simulink model "first_3phase_multilevel"  (R2015a)
settings: Solver=ode45  StartTime=0.02  StopTime=0.04  RelTol=1e-3
libraries: powerlib x95, powerlib_meascontrol x50, simulink x48, dspstat3 x2
(part 1 of 2)
settings Model: Creator=yahya  LastModifiedBy=Yahya

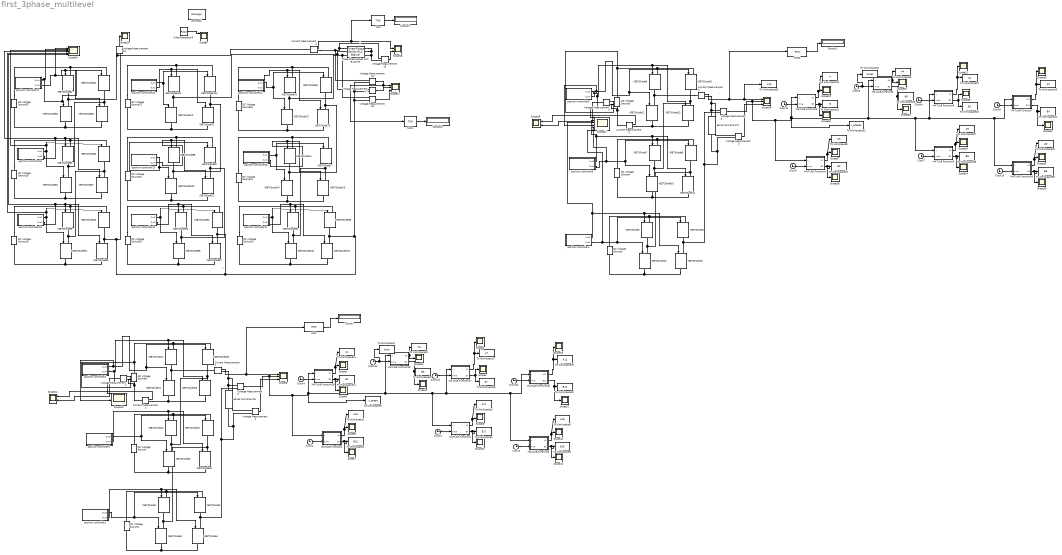
== system first_3phase_multilevel ==
  note: i
  note: n
  note: i
  note: i
  Clock{1..11,19..21} (14 alike) : Clock
  Current Measurement{1..5} (5 alike) : powerlib/Measurements/Current Measurement  PhasorSimulation=off  OutputType=Complex  PSBequivalent=0
  DC Voltage Source{1,3..5,7..8,18..26} (15 alike) : powerlib/Electrical Sources/DC Voltage Source  Amplitude=100  Measurements=None
  Display{,1..3} (4 alike) : Display
  IGBT/Diode{1..16,22..29,69..104} (60 alike) : powerlib/Power Electronics/IGBT//Diode  Ron=1e-3  Rs=1e5  Cs=inf  Measurements=off
  MATLAB Function1 : MATLAB Function  TreatAsAtomicUnit=on
  MATLAB Function10 : MATLAB Function  TreatAsAtomicUnit=on
  MATLAB Function16 : MATLAB Function  TreatAsAtomicUnit=on
  MATLAB Function17 : MATLAB Function  TreatAsAtomicUnit=on
  MATLAB Function18 : MATLAB Function  TreatAsAtomicUnit=on
  MATLAB Function19 : MATLAB Function  TreatAsAtomicUnit=on
  MATLAB Function2 : MATLAB Function  TreatAsAtomicUnit=on
  MATLAB Function3 : MATLAB Function  TreatAsAtomicUnit=on
  MATLAB Function4 : MATLAB Function  TreatAsAtomicUnit=on
  MATLAB Function5 : MATLAB Function  TreatAsAtomicUnit=on
  MATLAB Function6 : MATLAB Function  TreatAsAtomicUnit=on
  MATLAB Function7 : MATLAB Function  TreatAsAtomicUnit=on
  MATLAB Function8 : MATLAB Function  TreatAsAtomicUnit=on
  MATLAB Function9 : MATLAB Function  TreatAsAtomicUnit=on
  Pulse Generator3 : DiscretePulseGenerator  PulseType=Time based  Amplitude=0.8  Period=0.00001  PulseWidth=50
  RMS : dspstat3/RMS  run=off  reset_popup=None  InputProcessing=Columns as channels (frame based)  directionMode=Each column  dimension=1  treatSBRowAsCol=off
  RMS1 : dspstat3/RMS  run=off  reset_popup=None  InputProcessing=Columns as channels (frame based)  directionMode=Each column  dimension=1  treatSBRowAsCol=off
  Scope{1..4,6..8,10..12,15,19..26,29..35,37..39} (29 alike) : Scope
      Scope1 settings: TimeRange=0.2  YMin=190  YMax=400  SaveName=ScopeData6
      Scope10 settings: TimeRange=0.2  YMin=190  YMax=400  SaveName=ScopeData12
      Scope11 settings: TimeRange=0.2  YMin=190  YMax=400  SaveName=ScopeData14
      Scope12 settings: TimeRange=0.2  YMin=190  YMax=400  SaveName=ScopeData24
      Scope15 settings: TimeRange=0.2  YMin=190  YMax=400  SaveName=ScopeData27
      Scope19 settings: SaveName=ScopeData17
      Scope2 settings: TimeRange=0.2  YMin=190  YMax=400  SaveName=ScopeData7
      Scope20 settings: TimeRange=0.2  YMin=190  YMax=400  SaveName=ScopeData20
      Scope21 settings: TimeRange=0.2  YMin=190  YMax=400  SaveName=ScopeData21
      Scope22 settings: TimeRange=0.2  YMin=190  YMax=400  SaveName=ScopeData22
      Scope23 settings: TimeRange=0.2  YMin=190  YMax=400  SaveName=ScopeData23
      Scope24 settings: TimeRange=0.2  YMin=190  YMax=400  SaveName=ScopeData28
      Scope25 settings: TimeRange=0.2  YMin=190  YMax=400  SaveName=ScopeData29
      Scope26 settings: TimeRange=0.2  YMin=190  YMax=400  SaveName=ScopeData30
      Scope29 settings: TimeRange=0.2  YMin=190  YMax=400  SaveName=ScopeData33
      Scope3 settings: TimeRange=0.2  YMin=190  YMax=400  SaveName=ScopeData9
      Scope30 settings: TimeRange=0.2  YMin=190  YMax=400  SaveName=ScopeData34
      Scope31 settings: TimeRange=0.2  YMin=190  YMax=400  SaveName=ScopeData35
      Scope32 settings: TimeRange=0.2  YMin=190  YMax=400  SaveName=ScopeData36
      Scope33 settings: TimeRange=0.2  YMin=190  YMax=400  SaveName=ScopeData37
      Scope34 settings: TimeRange=0.2  YMin=190  YMax=400  SaveName=ScopeData38
      Scope35 settings: TimeRange=0.2  YMin=190  YMax=400  SaveName=ScopeData39
      Scope37 settings: TimeRange=0.2  YMin=190  YMax=400  SaveName=ScopeData41
      Scope38 settings: TimeRange=0.2  YMin=190  YMax=400  SaveName=ScopeData42
      Scope39 settings: TimeRange=0.2  YMin=190  YMax=400  SaveName=ScopeData43
      Scope4 settings: TimeRange=0.2  YMin=190  YMax=400  SaveName=ScopeData19
      Scope6 settings: TimeRange=0.2  YMin=190  YMax=400  SaveName=ScopeData10
      Scope7 settings: TimeRange=0.2  YMin=190  YMax=400  SaveName=ScopeData11
      Scope8 settings: TimeRange=0.2  YMin=190  YMax=400  SaveName=ScopeData13
  Scope13 : Scope  NumInputPorts=6
      settings: TimeRange=0.2  YMin=190~-5~-5~-5~-5~-5  YMax=400~5~5~5~5~5  SaveName=ScopeData25
  Scope14 : Scope  NumInputPorts=2
      settings: TimeRange=0.2  YMin=190~-5  YMax=400~5  SaveName=ScopeData26
  Scope16 : Scope  NumInputPorts=6
      settings: YMin=-5~-5~-5~-5~-5~-5  YMax=5~5~5~5~5~5  SaveName=ScopeData8
  Scope17 : Scope  NumInputPorts=3
      settings: TimeRange=0.02  YMin=-5~-5~-5  YMax=5~5~5  SaveName=ScopeData15
  Scope18 : Scope  NumInputPorts=2
      settings: TimeRange=1  YMin=-400~-400  YMax=400~400  SaveName=ScopeData16
  Scope27 : Scope  NumInputPorts=6
      settings: TimeRange=0.2  YMin=190~-5~-5~-5~-5~-5  YMax=400~5~5~5~5~5  SaveName=ScopeData31
  Scope28 : Scope  NumInputPorts=2
      settings: TimeRange=0.2  YMin=190~-5  YMax=400~5  SaveName=ScopeData32
  Scope36 : Scope  NumInputPorts=3
      settings: TimeRange=1  YMin=-400~-400~-5  YMax=400~400~5  SaveName=ScopeData40
  Scope5 : Scope  NumInputPorts=3
      settings: TimeRange=1  YMin=-400~-400~-5  YMax=400~400~5  SaveName=ScopeData3
  Scope9 : Scope  NumInputPorts=4
      settings: YMin=-5~-5~-5~-5  YMax=5~5~5~5  SaveName=ScopeData18
  Series RLC Branch1 : powerlib/Elements/Series RLC Branch  LConnTagsString=__new0  RConnTagsString=__new0  BranchType=R  Resistance=2000  Inductance=1e-5  SetiL0=off  InitialCurrent=0  Capacitance=1e-6  Setx0=off  InitialVoltage=0  Measurements=None
  Series RLC Branch5 : powerlib/Elements/Series RLC Branch  LConnTagsString=__new0  RConnTagsString=__new0  BranchType=R  Resistance=3000  Inductance=1e-5  SetiL0=off  InitialCurrent=0  Capacitance=1e-6  Setx0=off  InitialVoltage=0  Measurements=None
  THD : powerlib_meascontrol/Measurements/THD  Freq=50  Ts=0
  THD1 : powerlib_meascontrol/Measurements/THD  Freq=50  Ts=0
  Three-Phase Series RLC Branch3 : powerlib/Elements/Three-Phase Series RLC Branch  LConnTagsString=A|B|C  RConnTagsString=A|B|C  BranchType=RL  Resistance=1.405*2  Inductance=0.005839*2  Capacitance=1e-6  Measurements=Branch voltages
  To Workspace1 : ToWorkspace  VariableName=A13  SaveFormat=Timeseries  SampleTime=-1
  To Workspace10 : ToWorkspace  VariableName=A  SaveFormat=Timeseries  SampleTime=-1
  To Workspace11 : ToWorkspace  VariableName=A1  SaveFormat=Timeseries  SampleTime=-1
  To Workspace12 : ToWorkspace  VariableName=B  SaveFormat=Timeseries  SampleTime=-1
  To Workspace13 : ToWorkspace  VariableName=A2  SaveFormat=Timeseries  SampleTime=-1
  To Workspace14 : ToWorkspace  VariableName=B1  SaveFormat=Timeseries  SampleTime=-1
  To Workspace15 : ToWorkspace  VariableName=B2  SaveFormat=Timeseries  SampleTime=-1
  To Workspace16 : ToWorkspace  VariableName=A3  SaveFormat=Timeseries  SampleTime=-1
  To Workspace17 : ToWorkspace  VariableName=A7  SaveFormat=Timeseries  SampleTime=-1
  To Workspace18 : ToWorkspace  VariableName=B7  SaveFormat=Timeseries  SampleTime=-1
  To Workspace19 : ToWorkspace  VariableName=A11  SaveFormat=Timeseries  SampleTime=-1
  To Workspace2 : ToWorkspace  VariableName=B13  SaveFormat=Timeseries  SampleTime=-1
  To Workspace20 : ToWorkspace  VariableName=B11  SaveFormat=Timeseries  SampleTime=-1
  To Workspace21 : ToWorkspace  VariableName=A5  SaveFormat=Timeseries  SampleTime=-1
  To Workspace22 : ToWorkspace  VariableName=B5  SaveFormat=Timeseries  SampleTime=-1
  To Workspace23 : ToWorkspace  VariableName=B3  SaveFormat=Timeseries  SampleTime=-1
  To Workspace24 : ToWorkspace  VariableName=B4  SaveFormat=Timeseries  SampleTime=-1
  To Workspace25 : ToWorkspace  VariableName=A4  SaveFormat=Timeseries  SampleTime=-1
  To Workspace26 : ToWorkspace  VariableName=B6  SaveFormat=Timeseries  SampleTime=-1
  To Workspace27 : ToWorkspace  VariableName=A6  SaveFormat=Timeseries  SampleTime=-1
  To Workspace28 : ToWorkspace  VariableName=B8  SaveFormat=Timeseries  SampleTime=-1
  To Workspace29 : ToWorkspace  VariableName=A8  SaveFormat=Timeseries  SampleTime=-1
  To Workspace3 : ToWorkspace  VariableName=A17  SaveFormat=Timeseries  SampleTime=-1
  To Workspace30 : ToWorkspace  VariableName=B9  SaveFormat=Timeseries  SampleTime=-1
  To Workspace31 : ToWorkspace  VariableName=time1  SaveFormat=Timeseries  SampleTime=-1
  To Workspace32 : ToWorkspace  VariableName=v_phase1  SaveFormat=Timeseries  SampleTime=-1
  To Workspace33 : ToWorkspace  VariableName=A10  SaveFormat=Timeseries  SampleTime=-1
  To Workspace4 : ToWorkspace  VariableName=B17  SaveFormat=Timeseries  SampleTime=-1
  To Workspace5 : ToWorkspace  VariableName=A19  SaveFormat=Timeseries  SampleTime=-1
  To Workspace6 : ToWorkspace  VariableName=B19  SaveFormat=Timeseries  SampleTime=-1
  To Workspace7 : ToWorkspace  VariableName=time  SaveFormat=Timeseries  SampleTime=-1
  To Workspace8 : ToWorkspace  VariableName=v_phase  SaveFormat=Timeseries  SampleTime=-1
  To Workspace9 : ToWorkspace  VariableName=A9  SaveFormat=Timeseries  SampleTime=-1
  Voltage Measurement{1..6,15..19} (11 alike) : powerlib/Measurements/Voltage Measurement  PhasorSimulation=off  OutputType=Complex  PSBequivalent=0
  position controller1 : Subsystem
  position controller17 : Subsystem
  position controller18 : Subsystem
  position controller19 : Subsystem
  position controller2 : Subsystem
  position controller20 : Subsystem
  position controller21 : Subsystem
  position controller22 : Subsystem
  position controller23 : Subsystem
  position controller24 : Subsystem
  position controller25 : Subsystem
  position controller3 : Subsystem
  position controller4 : Subsystem
  position controller5 : Subsystem
  position controller6 : Subsystem
  powergui : powerlib/powergui  Priority=1  SimulationMode=Continuous  SolverType=Tustin/Backward Euler (TBE)  SampleTime=50e-6  frequency=60  SPID=off  DisableSnubberDevices=off  DisableRonSwitches=off  DisableVfSwitches=off  SwTol=0  DisplayEquations=off  Interpol=off  methode=off  Ts=100  FunctionMessages=off  echomessages=off  HookPort=off  EnableUseOfTLC=off  x0status=blocks  frequencyindice=0  Pbase=100e6  ErrMax=1e-4  Iterations=50  UnitsV=kV  UnitsW=MW  buscounter=0  RestoreLinks=warning  ResistiveCurrentMeasurement=off  Frange=[0:2:500]  Ylog=off  Xlog=on  ShowGrid=off  save=off  variable=ZData  structure=0  ZoomFFT=off  StartTime=0.0  cycles=1  DisplayStyle=1  fundamental=60  FreqAxis=off  MaxFrequency=1000  frequencyindicesteady=1  RmsSteady=1  display=off
  wires:
  position controller2/2(Out4) -> Scope13/1, IGBT/Diode28/1, IGBT/Diode24/1
  position controller2/1(Out3) -> Scope13/4, IGBT/Diode26/1, IGBT/Diode27/1
  position controller3/2(Out4) -> IGBT/Diode29/1, IGBT/Diode22/1
  position controller3/1(Out3) -> IGBT/Diode23/1, IGBT/Diode25/1
  Current Measurement1/1 -> RMS/1, Scope5/1
  Voltage Measurement4/1 -> Scope5/3
  position controller17/2(Out2) -> Scope16/1, IGBT/Diode86/1, IGBT/Diode82/1
  Pulse Generator3/1 -> Scope9/1
  Current Measurement4/1 -> THD/1, Scope18/1
  position controller17/1(Out1) -> Scope16/2, IGBT/Diode85/1, IGBT/Diode84/1
  position controller18/2(Out2) -> Scope16/4, IGBT/Diode87/1, IGBT/Diode69/1
  position controller18/1(Out1) -> IGBT/Diode83/1, Scope16/3, IGBT/Diode80/1
  position controller22/2(Out2) -> IGBT/Diode71/1, IGBT/Diode102/1
  position controller22/1(Out1) -> IGBT/Diode70/1, IGBT/Diode104/1
  position controller23/2(Out2) -> IGBT/Diode72/1, IGBT/Diode88/1
  position controller23/1(Out1) -> IGBT/Diode103/1, IGBT/Diode92/1
  position controller24/2(Out2) -> IGBT/Diode74/1, IGBT/Diode78/1
  position controller24/1(Out1) -> IGBT/Diode81/1, IGBT/Diode73/1
  position controller25/2(Out2) -> IGBT/Diode75/1, IGBT/Diode76/1
  position controller25/1(Out1) -> IGBT/Diode79/1, IGBT/Diode77/1
  Voltage Measurement19/1 -> Scope19/1
  Voltage Measurement15/1 -> Scope18/2
  Voltage Measurement16/1 -> Scope17/1, THD1/1
  Voltage Measurement17/1 -> Scope17/2
  Voltage Measurement18/1 -> Scope17/3
  position controller19/2(Out2) -> Scope16/6, IGBT/Diode93/1, IGBT/Diode89/1
  position controller19/1(Out1) -> IGBT/Diode91/1, Scope16/5, IGBT/Diode90/1
  position controller20/2(Out2) -> IGBT/Diode97/1, IGBT/Diode94/1
  position controller20/1(Out1) -> IGBT/Diode96/1, IGBT/Diode95/1
  position controller21/2(Out2) -> IGBT/Diode101/1, IGBT/Diode98/1
  position controller21/1(Out1) -> IGBT/Diode100/1, IGBT/Diode99/1
  position controller1/2(Out4) -> IGBT/Diode4/1, IGBT/Diode1/1
  position controller1/1(Out3) -> IGBT/Diode3/1, IGBT/Diode2/1
  Clock4/1 -> MATLAB Function16/2(time)
  MATLAB Function16/1(A1) -> To Workspace11/1, Scope2/1
  MATLAB Function16/2(B1) -> Scope3/1, To Workspace14/1
  Clock19/1 -> MATLAB Function17/2(time)
  MATLAB Function17/1(A7) -> Scope1/1, To Workspace17/1
  MATLAB Function17/2(B7) -> To Workspace18/1, Scope4/1
  Clock20/1 -> MATLAB Function18/2(time)
  MATLAB Function18/1(A11) -> Scope20/1, To Workspace19/1
  MATLAB Function18/2(B11) -> Scope21/1, To Workspace20/1
  MATLAB Function19/1(A5) -> Scope22/1, To Workspace21/1
  MATLAB Function19/2(B5) -> Scope23/1, To Workspace22/1
  Clock1/1 -> MATLAB Function1/2(time)
  MATLAB Function1/1(A1) -> To Workspace1/1, Scope6/1
  MATLAB Function1/2(B1) -> Scope7/1, To Workspace2/1
  Clock2/1 -> MATLAB Function2/2(time)
  MATLAB Function2/1(A1) -> To Workspace3/1, Scope8/1
  MATLAB Function2/2(B1) -> Scope10/1, To Workspace4/1
  Clock3/1 -> MATLAB Function3/2(time)
  MATLAB Function3/1(A1) -> To Workspace5/1, Scope12/1
  MATLAB Function3/2(B1) -> Scope11/1, To Workspace6/1
  Voltage Measurement5/1 -> MATLAB Function1/1(u), MATLAB Function2/1(u), MATLAB Function3/1(u), MATLAB Function18/1(u), MATLAB Function17/1(u), MATLAB Function19/1(u), To Workspace8/1, MATLAB Function16/1(u), Scope5/2
  Clock21/1 -> To Workspace7/1, MATLAB Function19/2(time)
  Current Measurement2/1 -> Scope14/1
  Voltage Measurement1/1 -> Scope14/2
  RMS/1 -> Display/1
  position controller5/1(Out3) -> Scope27/1, IGBT/Diode13/1, IGBT/Diode9/1
  position controller5/2(Out4) -> Scope27/4, IGBT/Diode11/1, IGBT/Diode12/1
  position controller6/1(Out3) -> Scope27/2, IGBT/Diode14/1, IGBT/Diode7/1
  position controller6/2(Out4) -> Scope27/5, IGBT/Diode8/1, IGBT/Diode10/1
  Current Measurement3/1 -> RMS1/1, To Workspace33/1, Scope36/1
  Voltage Measurement3/1 -> Scope36/3
  position controller4/1(Out3) -> Scope27/3, IGBT/Diode16/1, IGBT/Diode5/1
  position controller4/2(Out4) -> Scope27/6, IGBT/Diode15/1, IGBT/Diode6/1
  Clock11/1 -> MATLAB Function5/2(time)
  MATLAB Function5/1(A1) -> To Workspace10/1, Scope29/1
  MATLAB Function5/2(B1) -> Scope34/1, To Workspace12/1
  Clock6/1 -> MATLAB Function6/2(time)
  MATLAB Function6/1(A7) -> Scope15/1, To Workspace13/1
  MATLAB Function6/2(B7) -> To Workspace15/1, Scope35/1
  Clock8/1 -> MATLAB Function7/2(time)
  MATLAB Function7/1(A11) -> Scope30/1, To Workspace16/1
  MATLAB Function7/2(B11) -> Scope31/1, To Workspace24/1
  MATLAB Function8/1(A5) -> Scope32/1, To Workspace25/1
  MATLAB Function8/2(B5) -> Scope33/1, To Workspace26/1
  Clock5/1 -> MATLAB Function4/2(time)
  MATLAB Function4/1(A1) -> To Workspace9/1, Scope37/1
  MATLAB Function4/2(B1) -> Scope38/1, To Workspace23/1
  Clock7/1 -> MATLAB Function9/2(time)
  MATLAB Function9/1(A1) -> To Workspace27/1, Scope39/1
  MATLAB Function9/2(B1) -> Scope24/1, To Workspace28/1
  Clock10/1 -> MATLAB Function10/2(time)
  MATLAB Function10/1(A1) -> To Workspace29/1, Scope26/1
  MATLAB Function10/2(B1) -> Scope25/1, To Workspace30/1
  Voltage Measurement6/1 -> MATLAB Function4/1(u), MATLAB Function9/1(u), MATLAB Function10/1(u), MATLAB Function7/1(u), MATLAB Function6/1(u), MATLAB Function8/1(u), To Workspace32/1, MATLAB Function5/1(u), Scope36/2
  Clock9/1 -> To Workspace31/1, MATLAB Function8/2(time)
  Current Measurement5/1 -> Scope28/1
  Voltage Measurement2/1 -> Scope28/2
  RMS1/1 -> Display1/1
  THD/1 -> Display2/1
  THD1/1 -> Display3/1
  connections:
  IGBT/Diode26/LConn1 -- IGBT/Diode24/LConn1 -- DC Voltage Source8/RConn1 -- Voltage Measurement1/LConn2
  IGBT/Diode28/RConn1 -- Current Measurement2/RConn1 -- IGBT/Diode27/RConn1
  IGBT/Diode24/RConn1 -- IGBT/Diode27/LConn1 -- Current Measurement1/LConn1
  DC Voltage Source7/RConn1 -- IGBT/Diode23/LConn1 -- IGBT/Diode22/LConn1
  DC Voltage Source7/LConn1 -- IGBT/Diode29/RConn1 -- IGBT/Diode25/RConn1
  IGBT/Diode22/RConn1 -- IGBT/Diode25/LConn1 -- IGBT/Diode28/LConn1 -- IGBT/Diode26/RConn1
  IGBT/Diode3/LConn1 -- IGBT/Diode29/LConn1 -- IGBT/Diode23/RConn1 -- IGBT/Diode1/RConn1
  Voltage Measurement5/LConn1 -- Series RLC Branch5/LConn1 -- Voltage Measurement4/LConn1 -- Current Measurement1/RConn1
  DC Voltage Source25/RConn1 -- IGBT/Diode84/LConn1 -- IGBT/Diode82/LConn1
  DC Voltage Source25/LConn1 -- IGBT/Diode85/RConn1 -- IGBT/Diode86/RConn1
  IGBT/Diode84/RConn1 -- IGBT/Diode86/LConn1 -- IGBT/Diode69/RConn1 -- IGBT/Diode83/LConn1
  DC Voltage Source18/RConn1 -- IGBT/Diode80/LConn1 -- IGBT/Diode69/LConn1
  DC Voltage Source18/LConn1 -- IGBT/Diode87/RConn1 -- IGBT/Diode83/RConn1
  DC Voltage Source23/RConn1 -- IGBT/Diode104/LConn1 -- IGBT/Diode102/LConn1
  DC Voltage Source23/LConn1 -- IGBT/Diode71/RConn1 -- IGBT/Diode70/RConn1
  Voltage Measurement17/LConn1 -- Three-Phase Series RLC Branch3/LConn2 -- IGBT/Diode102/RConn1 -- IGBT/Diode70/LConn1
  IGBT/Diode92/LConn1 -- DC Voltage Source22/RConn1 -- IGBT/Diode88/LConn1
  DC Voltage Source22/LConn1 -- IGBT/Diode72/RConn1 -- IGBT/Diode103/RConn1
  IGBT/Diode88/RConn1 -- IGBT/Diode103/LConn1 -- IGBT/Diode71/LConn1 -- IGBT/Diode104/RConn1
  DC Voltage Source26/RConn1 -- IGBT/Diode81/LConn1 -- IGBT/Diode78/LConn1
  DC Voltage Source26/LConn1 -- IGBT/Diode74/RConn1 -- IGBT/Diode73/RConn1
  DC Voltage Source24/RConn1 -- IGBT/Diode77/LConn1 -- IGBT/Diode76/LConn1
  DC Voltage Source24/LConn1 -- IGBT/Diode75/RConn1 -- IGBT/Diode79/RConn1
  IGBT/Diode74/LConn1 -- IGBT/Diode81/RConn1 -- IGBT/Diode76/RConn1 -- IGBT/Diode79/LConn1
  IGBT/Diode73/LConn1 -- IGBT/Diode78/RConn1 -- Three-Phase Series RLC Branch3/LConn3 -- Voltage Measurement18/LConn1
  IGBT/Diode82/RConn1 -- IGBT/Diode85/LConn1 -- Current Measurement4/LConn1 -- Voltage Measurement19/LConn1
  Three-Phase Series RLC Branch3/LConn1 -- Voltage Measurement15/LConn1 -- Voltage Measurement16/LConn1 -- Current Measurement4/RConn1
  Three-Phase Series RLC Branch3/RConn1 -- Three-Phase Series RLC Branch3/RConn2 -- Three-Phase Series RLC Branch3/RConn3 -- Voltage Measurement15/LConn2
  IGBT/Diode89/RConn1 -- IGBT/Diode91/LConn1 -- IGBT/Diode80/RConn1 -- IGBT/Diode87/LConn1
  IGBT/Diode94/RConn1 -- IGBT/Diode96/LConn1 -- IGBT/Diode92/RConn1 -- IGBT/Diode72/LConn1
  IGBT/Diode98/RConn1 -- IGBT/Diode100/LConn1 -- IGBT/Diode77/RConn1 -- IGBT/Diode75/LConn1
  DC Voltage Source19/RConn1 -- IGBT/Diode90/LConn1 -- IGBT/Diode89/LConn1
  DC Voltage Source19/LConn1 -- IGBT/Diode93/RConn1 -- IGBT/Diode91/RConn1
  DC Voltage Source20/RConn1 -- IGBT/Diode95/LConn1 -- IGBT/Diode94/LConn1
  DC Voltage Source20/LConn1 -- IGBT/Diode97/RConn1 -- IGBT/Diode96/RConn1
  DC Voltage Source21/RConn1 -- IGBT/Diode99/LConn1 -- IGBT/Diode98/LConn1
  DC Voltage Source21/LConn1 -- IGBT/Diode101/RConn1 -- IGBT/Diode100/RConn1
  IGBT/Diode93/LConn1 -- IGBT/Diode90/RConn1 -- Voltage Measurement19/LConn2 -- Voltage Measurement16/LConn2 -- Voltage Measurement17/LConn2 -- Voltage Measurement18/LConn2 -- IGBT/Diode99/RConn1 -- IGBT/Diode101/LConn1 -- IGBT/Diode95/RConn1 -- IGBT/Diode97/LConn1
  IGBT/Diode1/LConn1 -- DC Voltage Source1/RConn1 -- IGBT/Diode2/LConn1
  IGBT/Diode3/RConn1 -- DC Voltage Source1/LConn1 -- IGBT/Diode4/RConn1
  Voltage Measurement4/LConn2 -- IGBT/Diode4/LConn1 -- IGBT/Diode2/RConn1 -- Voltage Measurement5/LConn2 -- Series RLC Branch5/RConn1
  DC Voltage Source8/LConn1 -- Current Measurement2/LConn1 -- Voltage Measurement1/LConn1
  IGBT/Diode9/LConn1 -- DC Voltage Source5/RConn1 -- Voltage Measurement2/LConn2 -- IGBT/Diode11/LConn1
  IGBT/Diode12/RConn1 -- IGBT/Diode13/RConn1 -- Current Measurement5/RConn1
  Current Measurement3/LConn1 -- IGBT/Diode9/RConn1 -- IGBT/Diode12/LConn1
  IGBT/Diode7/LConn1 -- DC Voltage Source4/RConn1 -- IGBT/Diode8/LConn1
  IGBT/Diode10/RConn1 -- DC Voltage Source4/LConn1 -- IGBT/Diode14/RConn1
  IGBT/Diode11/RConn1 -- IGBT/Diode13/LConn1 -- IGBT/Diode7/RConn1 -- IGBT/Diode10/LConn1
  IGBT/Diode5/RConn1 -- IGBT/Diode15/LConn1 -- IGBT/Diode14/LConn1 -- IGBT/Diode8/RConn1
  Current Measurement3/RConn1 -- Voltage Measurement3/LConn1 -- Voltage Measurement6/LConn1 -- Series RLC Branch1/LConn1
  IGBT/Diode6/LConn1 -- IGBT/Diode5/LConn1 -- DC Voltage Source3/RConn1
  IGBT/Diode16/RConn1 -- IGBT/Diode15/RConn1 -- DC Voltage Source3/LConn1
  Series RLC Branch1/RConn1 -- Voltage Measurement3/LConn2 -- IGBT/Diode16/LConn1 -- IGBT/Diode6/RConn1 -- Voltage Measurement6/LConn2
  Voltage Measurement2/LConn1 -- DC Voltage Source5/LConn1 -- Current Measurement5/LConn1

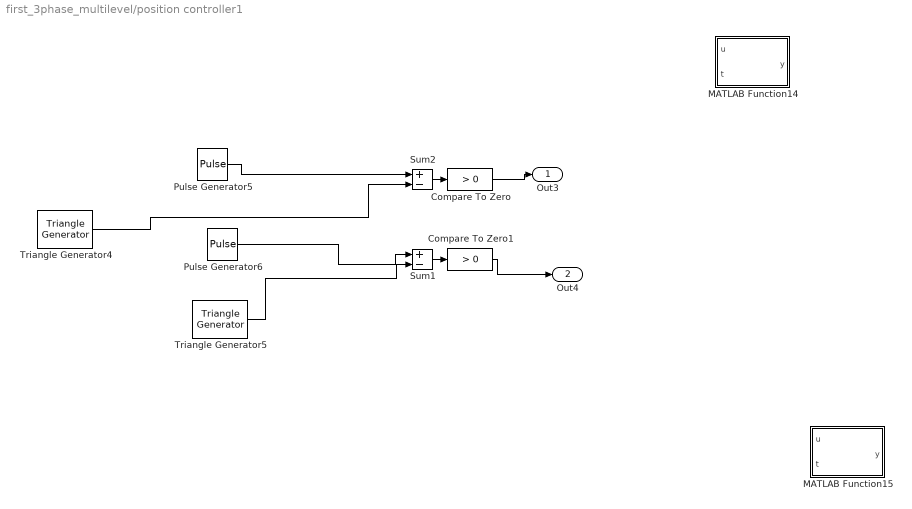
== system first_3phase_multilevel/position controller1 ==
  Compare To Zero : simulink/Logic and Bit Operations/Compare To Zero  relop=>  OutDataTypeStr=boolean  ZeroCross=off
  Compare To Zero1 : simulink/Logic and Bit Operations/Compare To Zero  relop=>  OutDataTypeStr=boolean  ZeroCross=off
  MATLAB Function14 : MATLAB Function  TreatAsAtomicUnit=on
  MATLAB Function15 : MATLAB Function  TreatAsAtomicUnit=on
  Pulse Generator5 : DiscretePulseGenerator  PulseType=Time based  Amplitude=0.138082553598467  Period=0.02  PulseWidth=50.001
  Pulse Generator6 : DiscretePulseGenerator  PulseType=Time based  Amplitude=0.138082553598467  Period=0.02  PulseWidth=50.001  PhaseDelay=0.01
  Sum1 : Sum  Inputs=+-  OutDataTypeStr=double
  Sum2 : Sum  Inputs=+-  OutDataTypeStr=double
  Triangle Generator4 : powerlib_meascontrol/Pulse & Signal Generators/Triangle Generator  Freq=50  Phase=90  Ts=0
  Triangle Generator5 : powerlib_meascontrol/Pulse & Signal Generators/Triangle Generator  Freq=50  Phase=90+180  Ts=0
  Out3 : Outport
  Out4 : Outport  Port=2
  wires:
  Compare To Zero/1 -> Out3/1
  Compare To Zero1/1 -> Out4/1
  Triangle Generator4/1 -> Sum2/2
  Sum2/1 -> Compare To Zero/1
  Sum1/1 -> Compare To Zero1/1
  Pulse Generator5/1 -> Sum2/1
  Pulse Generator6/1 -> Sum1/1
  Triangle Generator5/1 -> Sum1/2

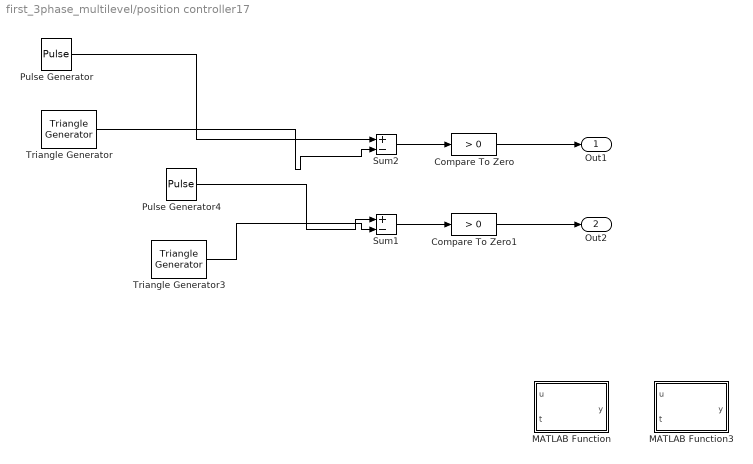
== system first_3phase_multilevel/position controller17 ==
  Compare To Zero : simulink/Logic and Bit Operations/Compare To Zero  relop=>  OutDataTypeStr=boolean  ZeroCross=off
  Compare To Zero1 : simulink/Logic and Bit Operations/Compare To Zero  relop=>  OutDataTypeStr=boolean  ZeroCross=off
  MATLAB Function : MATLAB Function  TreatAsAtomicUnit=on
  MATLAB Function3 : MATLAB Function  TreatAsAtomicUnit=on
  Pulse Generator : DiscretePulseGenerator  PulseType=Time based  Amplitude=0.9774  Period=0.02  PulseWidth=50
  Pulse Generator4 : DiscretePulseGenerator  PulseType=Time based  Amplitude=0.9774  Period=0.02  PulseWidth=50  PhaseDelay=0.01
  Sum1 : Sum  Inputs=+-  OutDataTypeStr=double
  Sum2 : Sum  Inputs=+-  OutDataTypeStr=double
  Triangle Generator : powerlib_meascontrol/Pulse & Signal Generators/Triangle Generator  Freq=50  Phase=90  Ts=0
  Triangle Generator3 : powerlib_meascontrol/Pulse & Signal Generators/Triangle Generator  Freq=50  Phase=90+180  Ts=0
  Out1 : Outport
  Out2 : Outport  Port=2
  wires:
  Compare To Zero/1 -> Out1/1
  Pulse Generator/1 -> Sum2/1
  Triangle Generator/1 -> Sum2/2
  Pulse Generator4/1 -> Sum1/1
  Triangle Generator3/1 -> Sum1/2
  Compare To Zero1/1 -> Out2/1
  Sum2/1 -> Compare To Zero/1
  Sum1/1 -> Compare To Zero1/1

== system first_3phase_multilevel/position controller18 ==
  Compare To Zero : simulink/Logic and Bit Operations/Compare To Zero  relop=>  OutDataTypeStr=boolean  ZeroCross=off
  Compare To Zero1 : simulink/Logic and Bit Operations/Compare To Zero  relop=>  OutDataTypeStr=boolean  ZeroCross=off
  Pulse Generator5 : DiscretePulseGenerator  PulseType=Time based  Amplitude=0.9502  Period=0.02  PulseWidth=50
  Pulse Generator6 : DiscretePulseGenerator  PulseType=Time based  Amplitude=0.9502  Period=0.02  PulseWidth=50  PhaseDelay=0.01
  Sum1 : Sum  Inputs=+-  OutDataTypeStr=double
  Sum2 : Sum  Inputs=+-  OutDataTypeStr=double
  Triangle Generator4 : powerlib_meascontrol/Pulse & Signal Generators/Triangle Generator  Freq=50  Phase=90  Ts=0
  Triangle Generator5 : powerlib_meascontrol/Pulse & Signal Generators/Triangle Generator  Freq=50  Phase=90+180  Ts=0
  Out1 : Outport
  Out2 : Outport  Port=2
  wires:
  Compare To Zero/1 -> Out1/1
  Compare To Zero1/1 -> Out2/1
  Pulse Generator5/1 -> Sum2/1
  Triangle Generator4/1 -> Sum2/2
  Pulse Generator6/1 -> Sum1/1
  Triangle Generator5/1 -> Sum1/2
  Sum2/1 -> Compare To Zero/1
  Sum1/1 -> Compare To Zero1/1

== system first_3phase_multilevel/position controller19 ==
  Compare To Zero : simulink/Logic and Bit Operations/Compare To Zero  relop=>  OutDataTypeStr=boolean  ZeroCross=off
  Compare To Zero1 : simulink/Logic and Bit Operations/Compare To Zero  relop=>  OutDataTypeStr=boolean  ZeroCross=off
  Pulse Generator5 : DiscretePulseGenerator  PulseType=Time based  Amplitude=0.5294  Period=0.02  PulseWidth=50
  Pulse Generator6 : DiscretePulseGenerator  PulseType=Time based  Amplitude=0.5294  Period=0.02  PulseWidth=50  PhaseDelay=0.01
  Sum1 : Sum  Inputs=+-  OutDataTypeStr=double
  Sum2 : Sum  Inputs=+-  OutDataTypeStr=double
  Triangle Generator4 : powerlib_meascontrol/Pulse & Signal Generators/Triangle Generator  Freq=50  Phase=90  Ts=0
  Triangle Generator5 : powerlib_meascontrol/Pulse & Signal Generators/Triangle Generator  Freq=50  Phase=90+180  Ts=0
  Out1 : Outport
  Out2 : Outport  Port=2
  wires:
  Compare To Zero/1 -> Out1/1
  Compare To Zero1/1 -> Out2/1
  Pulse Generator5/1 -> Sum2/1
  Triangle Generator4/1 -> Sum2/2
  Pulse Generator6/1 -> Sum1/1
  Triangle Generator5/1 -> Sum1/2
  Sum2/1 -> Compare To Zero/1
  Sum1/1 -> Compare To Zero1/1

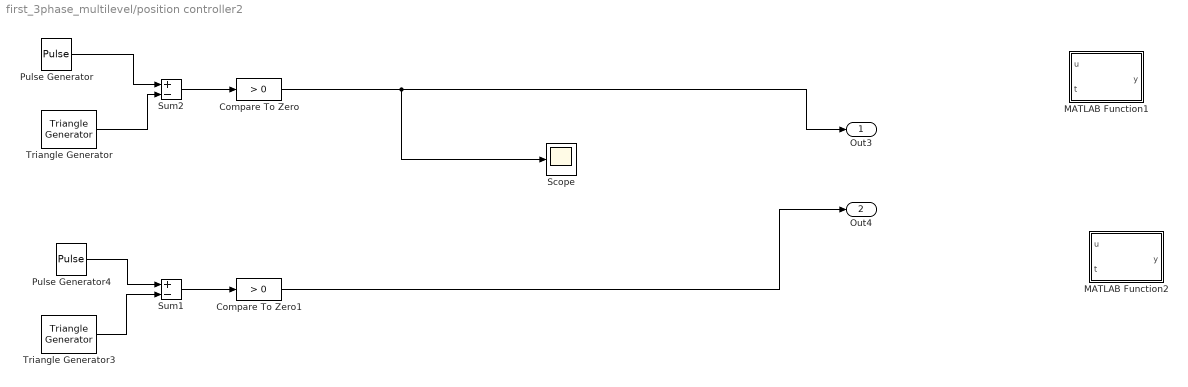
== system first_3phase_multilevel/position controller2 ==
  Compare To Zero : simulink/Logic and Bit Operations/Compare To Zero  relop=>  OutDataTypeStr=boolean  ZeroCross=off
  Compare To Zero1 : simulink/Logic and Bit Operations/Compare To Zero  relop=>  OutDataTypeStr=boolean  ZeroCross=off
  MATLAB Function1 : MATLAB Function  TreatAsAtomicUnit=on
  MATLAB Function2 : MATLAB Function  TreatAsAtomicUnit=on
  Pulse Generator : DiscretePulseGenerator  PulseType=Time based  Amplitude=0.638518973425229  Period=0.02  PulseWidth=50.001
  Pulse Generator4 : DiscretePulseGenerator  PulseType=Time based  Amplitude=0.638518973425229  Period=0.02  PulseWidth=50.001  PhaseDelay=0.01
  Scope : Scope
  Sum1 : Sum  Inputs=+-  OutDataTypeStr=double
  Sum2 : Sum  Inputs=+-  OutDataTypeStr=double
  Triangle Generator : powerlib_meascontrol/Pulse & Signal Generators/Triangle Generator  Freq=50  Phase=90  Ts=0
  Triangle Generator3 : powerlib_meascontrol/Pulse & Signal Generators/Triangle Generator  Freq=50  Phase=90+180  Ts=0
  Out3 : Outport
  Out4 : Outport  Port=2
  wires:
  Pulse Generator/1 -> Sum2/1
  Triangle Generator/1 -> Sum2/2
  Pulse Generator4/1 -> Sum1/1
  Triangle Generator3/1 -> Sum1/2
  Compare To Zero1/1 -> Out4/1
  Sum2/1 -> Compare To Zero/1
  Sum1/1 -> Compare To Zero1/1
  Compare To Zero/1 -> Scope/1, Out3/1

== system first_3phase_multilevel/position controller20 ==
  Compare To Zero : simulink/Logic and Bit Operations/Compare To Zero  relop=>  OutDataTypeStr=boolean  ZeroCross=off
  Compare To Zero1 : simulink/Logic and Bit Operations/Compare To Zero  relop=>  OutDataTypeStr=boolean  ZeroCross=off
  Pulse Generator5 : DiscretePulseGenerator  PulseType=Time based  Amplitude=0.5294  Period=0.02  PulseWidth=50
  Pulse Generator6 : DiscretePulseGenerator  PulseType=Time based  Amplitude=0.5294  Period=0.02  PulseWidth=50  PhaseDelay=0.01
  Sum1 : Sum  Inputs=+-  OutDataTypeStr=double
  Sum2 : Sum  Inputs=+-  OutDataTypeStr=double
  Triangle Generator4 : powerlib_meascontrol/Pulse & Signal Generators/Triangle Generator  Freq=50  Phase=90+240  Ts=0
  Triangle Generator5 : powerlib_meascontrol/Pulse & Signal Generators/Triangle Generator  Freq=50  Phase=90+180+240  Ts=0
  Out1 : Outport
  Out2 : Outport  Port=2
  wires:
  Compare To Zero/1 -> Out1/1
  Compare To Zero1/1 -> Out2/1
  Pulse Generator5/1 -> Sum2/1
  Triangle Generator4/1 -> Sum2/2
  Pulse Generator6/1 -> Sum1/1
  Triangle Generator5/1 -> Sum1/2
  Sum2/1 -> Compare To Zero/1
  Sum1/1 -> Compare To Zero1/1

== system first_3phase_multilevel/position controller21 ==
  Compare To Zero : simulink/Logic and Bit Operations/Compare To Zero  relop=>  OutDataTypeStr=boolean  ZeroCross=off
  Compare To Zero1 : simulink/Logic and Bit Operations/Compare To Zero  relop=>  OutDataTypeStr=boolean  ZeroCross=off
  Pulse Generator5 : DiscretePulseGenerator  PulseType=Time based  Amplitude=0.5294  Period=0.535476666666667  PulseWidth=50
  Pulse Generator6 : DiscretePulseGenerator  PulseType=Time based  Amplitude=0.5294  Period=0.02  PulseWidth=50  PhaseDelay=0.01
  Sum1 : Sum  Inputs=+-  OutDataTypeStr=double
  Sum2 : Sum  Inputs=+-  OutDataTypeStr=double
  Triangle Generator4 : powerlib_meascontrol/Pulse & Signal Generators/Triangle Generator  Freq=50  Phase=90+120  Ts=0
  Triangle Generator5 : powerlib_meascontrol/Pulse & Signal Generators/Triangle Generator  Freq=50  Phase=90+180+120  Ts=0
  Out1 : Outport
  Out2 : Outport  Port=2
  wires:
  Compare To Zero/1 -> Out1/1
  Compare To Zero1/1 -> Out2/1
  Pulse Generator5/1 -> Sum2/1
  Triangle Generator4/1 -> Sum2/2
  Pulse Generator6/1 -> Sum1/1
  Triangle Generator5/1 -> Sum1/2
  Sum2/1 -> Compare To Zero/1
  Sum1/1 -> Compare To Zero1/1

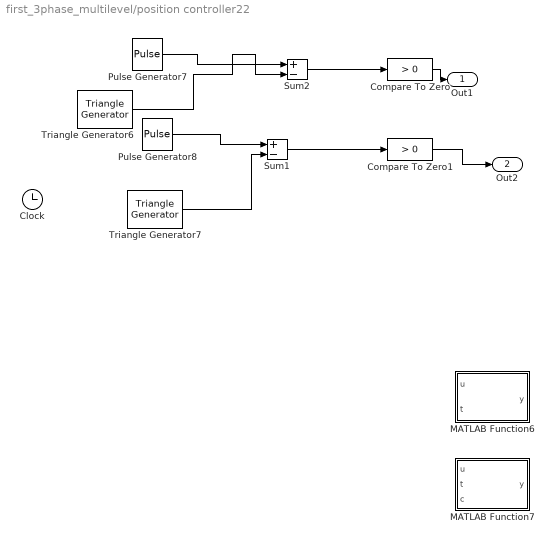
== system first_3phase_multilevel/position controller22 ==
  Clock : Clock
  Compare To Zero : simulink/Logic and Bit Operations/Compare To Zero  relop=>  OutDataTypeStr=boolean  ZeroCross=off
  Compare To Zero1 : simulink/Logic and Bit Operations/Compare To Zero  relop=>  OutDataTypeStr=boolean  ZeroCross=off
  MATLAB Function6 : MATLAB Function  TreatAsAtomicUnit=on
  MATLAB Function7 : MATLAB Function  TreatAsAtomicUnit=on
  Pulse Generator7 : DiscretePulseGenerator  PulseType=Time based  Amplitude=0.9774  Period=0.02  PulseWidth=50  PhaseDelay=0.00666
  Pulse Generator8 : DiscretePulseGenerator  PulseType=Time based  Amplitude=0.9774  Period=0.02  PulseWidth=50  PhaseDelay=0.01+0.00666
  Sum1 : Sum  Inputs=+-  OutDataTypeStr=double
  Sum2 : Sum  Inputs=+-  OutDataTypeStr=double
  Triangle Generator6 : powerlib_meascontrol/Pulse & Signal Generators/Triangle Generator  Freq=50  Phase=90+240  Ts=0
  Triangle Generator7 : powerlib_meascontrol/Pulse & Signal Generators/Triangle Generator  Freq=50  Phase=90+180+240  Ts=0
  Out1 : Outport
  Out2 : Outport  Port=2
  wires:
  Compare To Zero/1 -> Out1/1
  Compare To Zero1/1 -> Out2/1
  Triangle Generator6/1 -> Sum2/2
  Pulse Generator8/1 -> Sum1/1
  Pulse Generator7/1 -> Sum2/1
  Triangle Generator7/1 -> Sum1/2
  Sum2/1 -> Compare To Zero/1
  Sum1/1 -> Compare To Zero1/1

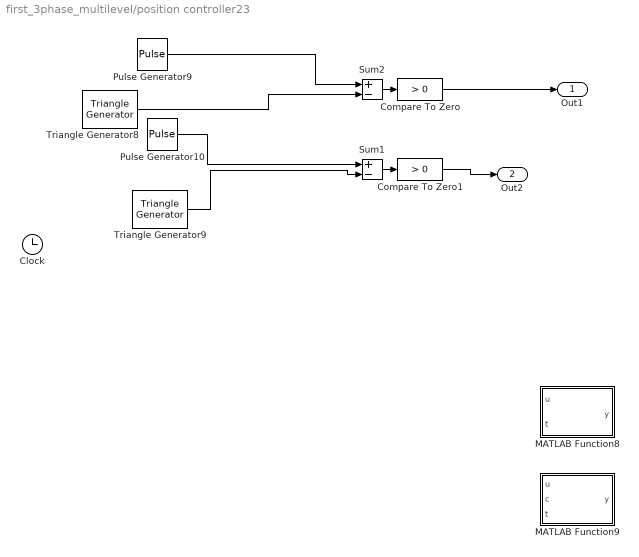
== system first_3phase_multilevel/position controller23 ==
  Clock : Clock
  Compare To Zero : simulink/Logic and Bit Operations/Compare To Zero  relop=>  OutDataTypeStr=boolean  ZeroCross=off
  Compare To Zero1 : simulink/Logic and Bit Operations/Compare To Zero  relop=>  OutDataTypeStr=boolean  ZeroCross=off
  MATLAB Function8 : MATLAB Function  TreatAsAtomicUnit=on
  MATLAB Function9 : MATLAB Function  TreatAsAtomicUnit=on
  Pulse Generator10 : DiscretePulseGenerator  PulseType=Time based  Amplitude=0.9502  Period=0.02  PulseWidth=50  PhaseDelay=0.01+0.00666
  Pulse Generator9 : DiscretePulseGenerator  PulseType=Time based  Amplitude=0.9502  Period=0.02  PulseWidth=50  PhaseDelay=0.00666
  Sum1 : Sum  Inputs=+-  OutDataTypeStr=double
  Sum2 : Sum  Inputs=+-  OutDataTypeStr=double
  Triangle Generator8 : powerlib_meascontrol/Pulse & Signal Generators/Triangle Generator  Freq=50  Phase=90+240  Ts=0
  Triangle Generator9 : powerlib_meascontrol/Pulse & Signal Generators/Triangle Generator  Freq=50  Phase=90+180+240  Ts=0
  Out1 : Outport
  Out2 : Outport  Port=2
  wires:
  Compare To Zero/1 -> Out1/1
  Triangle Generator8/1 -> Sum2/2
  Compare To Zero1/1 -> Out2/1
  Pulse Generator10/1 -> Sum1/1
  Triangle Generator9/1 -> Sum1/2
  Sum2/1 -> Compare To Zero/1
  Sum1/1 -> Compare To Zero1/1
  Pulse Generator9/1 -> Sum2/1

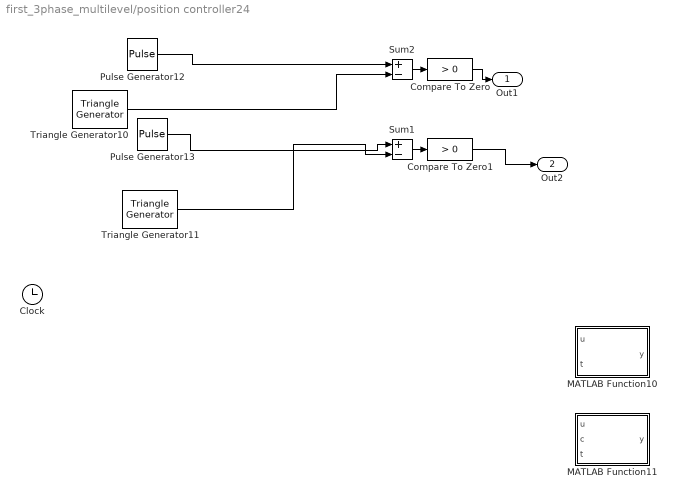
== system first_3phase_multilevel/position controller24 ==
  Clock : Clock
  Compare To Zero : simulink/Logic and Bit Operations/Compare To Zero  relop=>  OutDataTypeStr=boolean  ZeroCross=off
  Compare To Zero1 : simulink/Logic and Bit Operations/Compare To Zero  relop=>  OutDataTypeStr=boolean  ZeroCross=off
  MATLAB Function10 : MATLAB Function  TreatAsAtomicUnit=on
  MATLAB Function11 : MATLAB Function  TreatAsAtomicUnit=on
  Pulse Generator12 : DiscretePulseGenerator  PulseType=Time based  Amplitude=0.9774  Period=0.02  PulseWidth=50  PhaseDelay=0.00666*2
  Pulse Generator13 : DiscretePulseGenerator  PulseType=Time based  Amplitude=0.9774  Period=0.02  PulseWidth=50  PhaseDelay=0.01+0.00666*2
  Sum1 : Sum  Inputs=+-  OutDataTypeStr=double
  Sum2 : Sum  Inputs=+-  OutDataTypeStr=double
  Triangle Generator10 : powerlib_meascontrol/Pulse & Signal Generators/Triangle Generator  Freq=50  Phase=90+120  Ts=0
  Triangle Generator11 : powerlib_meascontrol/Pulse & Signal Generators/Triangle Generator  Freq=50  Phase=90+180+120  Ts=0
  Out1 : Outport
  Out2 : Outport  Port=2
  wires:
  Compare To Zero/1 -> Out1/1
  Compare To Zero1/1 -> Out2/1
  Triangle Generator10/1 -> Sum2/2
  Pulse Generator13/1 -> Sum1/1
  Triangle Generator11/1 -> Sum1/2
  Pulse Generator12/1 -> Sum2/1
  Sum2/1 -> Compare To Zero/1
  Sum1/1 -> Compare To Zero1/1

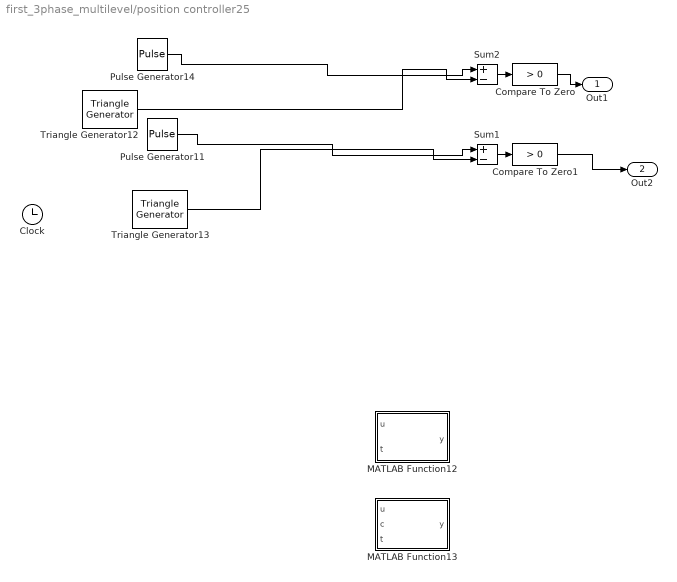
== system first_3phase_multilevel/position controller25 ==
  Clock : Clock
  Compare To Zero : simulink/Logic and Bit Operations/Compare To Zero  relop=>  OutDataTypeStr=boolean  ZeroCross=off
  Compare To Zero1 : simulink/Logic and Bit Operations/Compare To Zero  relop=>  OutDataTypeStr=boolean  ZeroCross=off
  MATLAB Function12 : MATLAB Function  TreatAsAtomicUnit=on
  MATLAB Function13 : MATLAB Function  TreatAsAtomicUnit=on
  Pulse Generator11 : DiscretePulseGenerator  PulseType=Time based  Amplitude=0.9502  Period=0.02  PulseWidth=50  PhaseDelay=0.01+0.00666*2
  Pulse Generator14 : DiscretePulseGenerator  PulseType=Time based  Amplitude=0.9502  Period=0.966211111111111  PulseWidth=50  PhaseDelay=0.00666*2
  Sum1 : Sum  Inputs=+-  OutDataTypeStr=double
  Sum2 : Sum  Inputs=+-  OutDataTypeStr=double
  Triangle Generator12 : powerlib_meascontrol/Pulse & Signal Generators/Triangle Generator  Freq=50  Phase=90+120  Ts=0
  Triangle Generator13 : powerlib_meascontrol/Pulse & Signal Generators/Triangle Generator  Freq=50  Phase=90+180+120  Ts=0
  Out1 : Outport
  Out2 : Outport  Port=2
  wires:
  Compare To Zero/1 -> Out1/1
  Compare To Zero1/1 -> Out2/1
  Pulse Generator14/1 -> Sum2/1
  Triangle Generator12/1 -> Sum2/2
  Pulse Generator11/1 -> Sum1/1
  Triangle Generator13/1 -> Sum1/2
  Sum2/1 -> Compare To Zero/1
  Sum1/1 -> Compare To Zero1/1

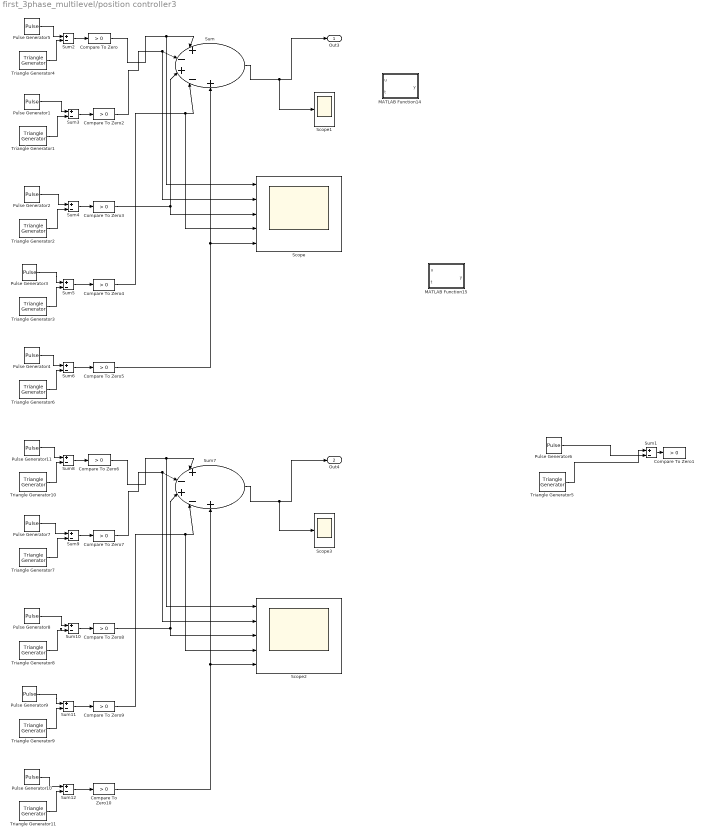
== system first_3phase_multilevel/position controller3 ==
  Compare To Zero{,1..10} (11 alike) : simulink/Logic and Bit Operations/Compare To Zero  relop=>  OutDataTypeStr=boolean  ZeroCross=off
  MATLAB Function14 : MATLAB Function  TreatAsAtomicUnit=on
  MATLAB Function15 : MATLAB Function  TreatAsAtomicUnit=on
  Pulse Generator1 : DiscretePulseGenerator  PulseType=Time based  Amplitude=0.348880750931017  Period=0.02  PulseWidth=50.001
  Pulse Generator10 : DiscretePulseGenerator  PulseType=Time based  Amplitude=0.377812988041322  Period=0.02  PulseWidth=50.001  PhaseDelay=0.01
  Pulse Generator11 : DiscretePulseGenerator  PulseType=Time based  Amplitude=0.289737494146879  Period=0.02  PulseWidth=.001  PhaseDelay=0.01
  Pulse Generator2 : DiscretePulseGenerator  PulseType=Time based  Amplitude=0.354483004927852  Period=0.02  PulseWidth=50.001
  Pulse Generator3 : DiscretePulseGenerator  PulseType=Time based  Amplitude=0.360085258924687  Period=0.02  PulseWidth=50.001
  Pulse Generator4 : DiscretePulseGenerator  PulseType=Time based  Amplitude=0.377812988041322  Period=0.02  PulseWidth=50.001
  Pulse Generator5 : DiscretePulseGenerator  PulseType=Time based  Amplitude=0.289737494146879  Period=0.02  PulseWidth=50.001
  Pulse Generator6 : DiscretePulseGenerator  PulseType=Time based  Amplitude=0.332  Period=0.02  PulseWidth=50  PhaseDelay=0.01
  Pulse Generator7 : DiscretePulseGenerator  PulseType=Time based  Amplitude=0.348880750931017  Period=0.02  PulseWidth=50.001  PhaseDelay=0.01
  Pulse Generator8 : DiscretePulseGenerator  PulseType=Time based  Amplitude=0.354483004927852  Period=0.02  PulseWidth=50.001  PhaseDelay=0.01
  Pulse Generator9 : DiscretePulseGenerator  PulseType=Time based  Amplitude=0.360085258924687  Period=0.02  PulseWidth=50.001  PhaseDelay=0.01
  Scope : Scope  NumInputPorts=5
      settings: YMin=-5~-5~-5~-5~-5  YMax=5~5~5~5~5
  Scope1 : Scope
      settings: SaveName=ScopeData2
  Scope2 : Scope  NumInputPorts=5
      settings: YMin=-5~-5~-5~-5~-5  YMax=5~5~5~5~5  SaveName=ScopeData4
  Scope3 : Scope
      settings: SaveName=ScopeData5
  Sum : Sum  Inputs=|+-+-+
  Sum{1..6,8..12} (11 alike) : Sum  Inputs=+-  OutDataTypeStr=double
  Sum7 : Sum  Inputs=|+-+-+
  Triangle Generator{1..4,6} (5 alike) : powerlib_meascontrol/Pulse & Signal Generators/Triangle Generator  Freq=50  Phase=90  Ts=0
  Triangle Generator{5,7..11} (6 alike) : powerlib_meascontrol/Pulse & Signal Generators/Triangle Generator  Freq=50  Phase=90+180  Ts=0
  Out3 : Outport
  Out4 : Outport  Port=2
  wires:
  Triangle Generator4/1 -> Sum2/2
  Sum2/1 -> Compare To Zero/1
  Sum1/1 -> Compare To Zero1/1
  Pulse Generator5/1 -> Sum2/1
  Pulse Generator6/1 -> Sum1/1
  Triangle Generator5/1 -> Sum1/2
  Triangle Generator1/1 -> Sum3/2
  Sum3/1 -> Compare To Zero2/1
  Pulse Generator1/1 -> Sum3/1
  Triangle Generator2/1 -> Sum4/2
  Sum4/1 -> Compare To Zero3/1
  Pulse Generator2/1 -> Sum4/1
  Triangle Generator3/1 -> Sum5/2
  Sum5/1 -> Compare To Zero4/1
  Pulse Generator3/1 -> Sum5/1
  Triangle Generator6/1 -> Sum6/2
  Sum6/1 -> Compare To Zero5/1
  Pulse Generator4/1 -> Sum6/1
  Compare To Zero/1 -> Scope/1, Sum/1
  Compare To Zero2/1 -> Scope/2, Sum/2
  Compare To Zero3/1 -> Sum/3, Scope/3
  Sum/1 -> Scope1/1, Out3/1
  Compare To Zero4/1 -> Scope/4, Sum/4
  Compare To Zero5/1 -> Scope/5, Sum/5
  Triangle Generator10/1 -> Sum8/2
  Sum8/1 -> Compare To Zero6/1
  Pulse Generator11/1 -> Sum8/1
  Triangle Generator7/1 -> Sum9/2
  Sum9/1 -> Compare To Zero7/1
  Pulse Generator7/1 -> Sum9/1
  Triangle Generator8/1 -> Sum10/2
  Sum10/1 -> Compare To Zero8/1
  Pulse Generator8/1 -> Sum10/1
  Triangle Generator9/1 -> Sum11/2
  Sum11/1 -> Compare To Zero9/1
  Pulse Generator9/1 -> Sum11/1
  Triangle Generator11/1 -> Sum12/2
  Sum12/1 -> Compare To Zero10/1
  Pulse Generator10/1 -> Sum12/1
  Compare To Zero6/1 -> Scope2/1, Sum7/1
  Compare To Zero7/1 -> Scope2/2, Sum7/2
  Compare To Zero8/1 -> Sum7/3, Scope2/3
  Sum7/1 -> Out4/1, Scope3/1
  Compare To Zero9/1 -> Scope2/4, Sum7/4
  Compare To Zero10/1 -> Scope2/5, Sum7/5

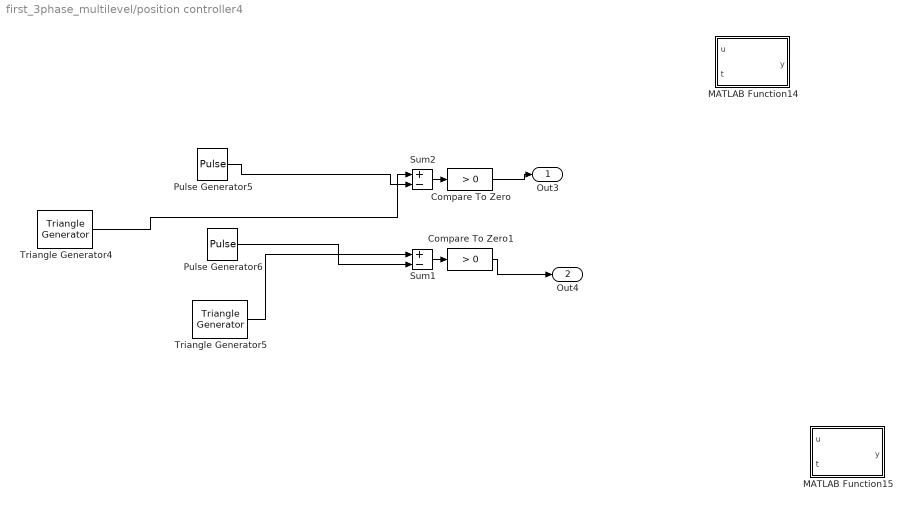
== system first_3phase_multilevel/position controller4 ==
  Compare To Zero : simulink/Logic and Bit Operations/Compare To Zero  relop=>  OutDataTypeStr=boolean  ZeroCross=off
  Compare To Zero1 : simulink/Logic and Bit Operations/Compare To Zero  relop=>  OutDataTypeStr=boolean  ZeroCross=off
  MATLAB Function14 : MATLAB Function  TreatAsAtomicUnit=on
  MATLAB Function15 : MATLAB Function  TreatAsAtomicUnit=on
  Pulse Generator5 : DiscretePulseGenerator  PulseType=Time based  Amplitude=0.137884444444444  Period=0.02  PulseWidth=50.001
  Pulse Generator6 : DiscretePulseGenerator  PulseType=Time based  Amplitude=0.137884444444444  Period=0.02  PulseWidth=50.001  PhaseDelay=0.01
  Sum1 : Sum  Inputs=+-  OutDataTypeStr=double
  Sum2 : Sum  Inputs=+-  OutDataTypeStr=double
  Triangle Generator4 : powerlib_meascontrol/Pulse & Signal Generators/Triangle Generator  Freq=50  Phase=90  Ts=0
  Triangle Generator5 : powerlib_meascontrol/Pulse & Signal Generators/Triangle Generator  Freq=50  Phase=90+180  Ts=0
  Out3 : Outport
  Out4 : Outport  Port=2
  wires:
  Compare To Zero/1 -> Out3/1
  Compare To Zero1/1 -> Out4/1
  Triangle Generator4/1 -> Sum2/1
  Sum2/1 -> Compare To Zero/1
  Sum1/1 -> Compare To Zero1/1
  Pulse Generator5/1 -> Sum2/2
  Pulse Generator6/1 -> Sum1/2
  Triangle Generator5/1 -> Sum1/1

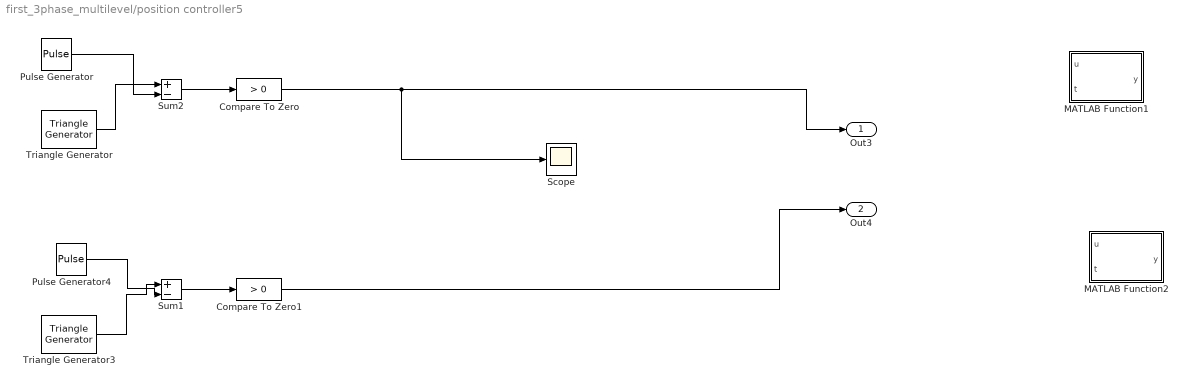
== system first_3phase_multilevel/position controller5 ==
  Compare To Zero : simulink/Logic and Bit Operations/Compare To Zero  relop=>  OutDataTypeStr=boolean  ZeroCross=off
  Compare To Zero1 : simulink/Logic and Bit Operations/Compare To Zero  relop=>  OutDataTypeStr=boolean  ZeroCross=off
  MATLAB Function1 : MATLAB Function  TreatAsAtomicUnit=on
  MATLAB Function2 : MATLAB Function  TreatAsAtomicUnit=on
  Pulse Generator : DiscretePulseGenerator  PulseType=Time based  Amplitude=0.638761111111111  Period=0.02  PulseWidth=50.001
  Pulse Generator4 : DiscretePulseGenerator  PulseType=Time based  Amplitude=0.638761111111111  Period=0.02  PulseWidth=50.001  PhaseDelay=0.01
  Scope : Scope
  Sum1 : Sum  Inputs=+-  OutDataTypeStr=double
  Sum2 : Sum  Inputs=+-  OutDataTypeStr=double
  Triangle Generator : powerlib_meascontrol/Pulse & Signal Generators/Triangle Generator  Freq=50  Phase=90  Ts=0
  Triangle Generator3 : powerlib_meascontrol/Pulse & Signal Generators/Triangle Generator  Freq=50  Phase=90+180  Ts=0
  Out3 : Outport
  Out4 : Outport  Port=2
  wires:
  Pulse Generator/1 -> Sum2/2
  Triangle Generator/1 -> Sum2/1
  Pulse Generator4/1 -> Sum1/2
  Triangle Generator3/1 -> Sum1/1
  Compare To Zero1/1 -> Out4/1
  Sum2/1 -> Compare To Zero/1
  Sum1/1 -> Compare To Zero1/1
  Compare To Zero/1 -> Scope/1, Out3/1

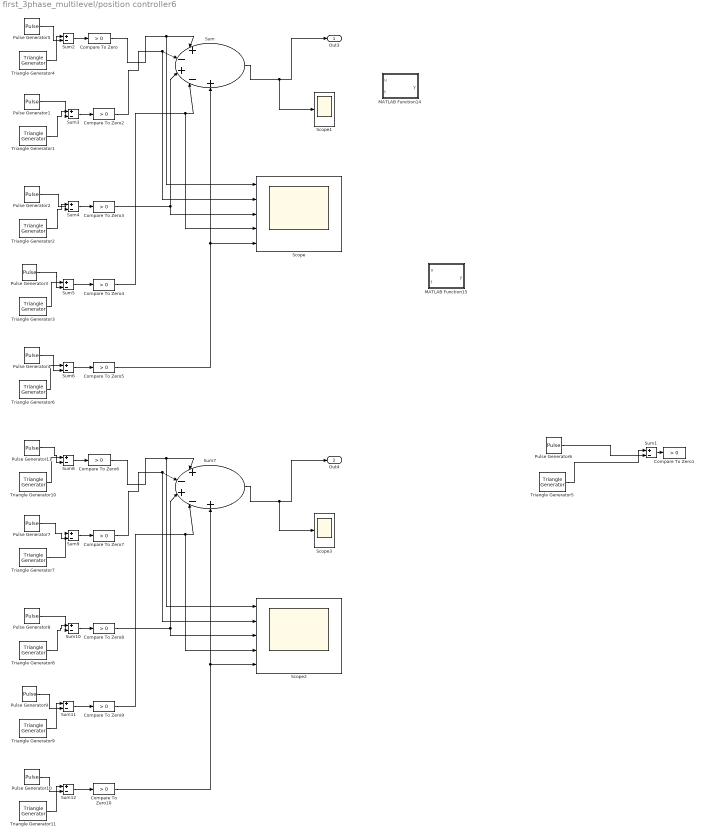
== system first_3phase_multilevel/position controller6 ==
  Compare To Zero{,1..10} (11 alike) : simulink/Logic and Bit Operations/Compare To Zero  relop=>  OutDataTypeStr=boolean  ZeroCross=off
  MATLAB Function14 : MATLAB Function  TreatAsAtomicUnit=on
  MATLAB Function15 : MATLAB Function  TreatAsAtomicUnit=on
  Pulse Generator1 : DiscretePulseGenerator  PulseType=Time based  Amplitude=0.359264444444444  Period=0.02  PulseWidth=50.001
  Pulse Generator10 : DiscretePulseGenerator  PulseType=Time based  Amplitude=0.633156666666667  Period=0.02  PulseWidth=50.001  PhaseDelay=0.01
  Pulse Generator11 : DiscretePulseGenerator  PulseType=Time based  Amplitude=0.295040000000000  Period=0.02  PulseWidth=50.001  PhaseDelay=0.01
  Pulse Generator2 : DiscretePulseGenerator  PulseType=Time based  Amplitude=0.386574444444444  Period=0.02  PulseWidth=50.001
  Pulse Generator3 : DiscretePulseGenerator  PulseType=Time based  Amplitude=0.627554444444444  Period=0.02  PulseWidth=50.001
  Pulse Generator4 : DiscretePulseGenerator  PulseType=Time based  Amplitude=0.633156666666667  Period=0.02  PulseWidth=50.001
  Pulse Generator5 : DiscretePulseGenerator  PulseType=Time based  Amplitude=0.295040000000000  Period=0.02  PulseWidth=50.001
  Pulse Generator6 : DiscretePulseGenerator  PulseType=Time based  Amplitude=0.332  Period=0.02  PulseWidth=50  PhaseDelay=0.01
  Pulse Generator7 : DiscretePulseGenerator  PulseType=Time based  Amplitude=0.359264444444444  Period=0.02  PulseWidth=50.001  PhaseDelay=0.01
  Pulse Generator8 : DiscretePulseGenerator  PulseType=Time based  Amplitude=0.386574444444444  Period=0.02  PulseWidth=50.001  PhaseDelay=0.01
  Pulse Generator9 : DiscretePulseGenerator  PulseType=Time based  Amplitude=0.627554444444444  Period=0.02  PulseWidth=50.001  PhaseDelay=0.01
  Scope : Scope  NumInputPorts=5
      settings: YMin=-5~-5~-5~-5~-5  YMax=5~5~5~5~5
  Scope1 : Scope
      settings: SaveName=ScopeData2
  Scope2 : Scope  NumInputPorts=5
      settings: YMin=-5~-5~-5~-5~-5  YMax=5~5~5~5~5  SaveName=ScopeData4
  Scope3 : Scope
      settings: SaveName=ScopeData5
  Sum : Sum  Inputs=|+-+-+
  Sum{1..6,8..12} (11 alike) : Sum  Inputs=+-  OutDataTypeStr=double
  Sum7 : Sum  Inputs=|+-+-+
  Triangle Generator{1..4,6} (5 alike) : powerlib_meascontrol/Pulse & Signal Generators/Triangle Generator  Freq=50  Phase=90  Ts=0
  Triangle Generator{5,7..11} (6 alike) : powerlib_meascontrol/Pulse & Signal Generators/Triangle Generator  Freq=50  Phase=90+180  Ts=0
  Out3 : Outport
  Out4 : Outport  Port=2
  wires:
  Triangle Generator4/1 -> Sum2/1
  Sum2/1 -> Compare To Zero/1
  Sum1/1 -> Compare To Zero1/1
  Pulse Generator5/1 -> Sum2/2
  Pulse Generator6/1 -> Sum1/1
  Triangle Generator5/1 -> Sum1/2
  Triangle Generator1/1 -> Sum3/1
  Sum3/1 -> Compare To Zero2/1
  Pulse Generator1/1 -> Sum3/2
  Triangle Generator2/1 -> Sum4/1
  Sum4/1 -> Compare To Zero3/1
  Pulse Generator2/1 -> Sum4/2
  Triangle Generator3/1 -> Sum5/1
  Sum5/1 -> Compare To Zero4/1
  Pulse Generator3/1 -> Sum5/2
  Triangle Generator6/1 -> Sum6/1
  Sum6/1 -> Compare To Zero5/1
  Pulse Generator4/1 -> Sum6/2
  Compare To Zero/1 -> Scope/1, Sum/1
  Compare To Zero2/1 -> Scope/2, Sum/2
  Compare To Zero3/1 -> Sum/3, Scope/3
  Sum/1 -> Scope1/1, Out3/1
  Compare To Zero4/1 -> Scope/4, Sum/4
  Compare To Zero5/1 -> Scope/5, Sum/5
  Triangle Generator10/1 -> Sum8/1
  Sum8/1 -> Compare To Zero6/1
  Pulse Generator11/1 -> Sum8/2
  Triangle Generator7/1 -> Sum9/1
  Sum9/1 -> Compare To Zero7/1
  Pulse Generator7/1 -> Sum9/2
  Triangle Generator8/1 -> Sum10/1
  Sum10/1 -> Compare To Zero8/1
  Pulse Generator8/1 -> Sum10/2
  Triangle Generator9/1 -> Sum11/1
  Sum11/1 -> Compare To Zero9/1
  Pulse Generator9/1 -> Sum11/2
  Triangle Generator11/1 -> Sum12/1
  Sum12/1 -> Compare To Zero10/1
  Pulse Generator10/1 -> Sum12/2
  Compare To Zero6/1 -> Scope2/1, Sum7/1
  Compare To Zero7/1 -> Scope2/2, Sum7/2
  Compare To Zero8/1 -> Sum7/3, Scope2/3
  Sum7/1 -> Out4/1, Scope3/1
  Compare To Zero9/1 -> Scope2/4, Sum7/4
  Compare To Zero10/1 -> Scope2/5, Sum7/5

== matlab function first_3phase_multilevel/position controller3/MATLAB Function14 ==
  data: u input; y output; t input
function y = fcn(u,t)
%#codegen
if t>u
    y = 1;
else
    y = 0;
end
end

== matlab function first_3phase_multilevel/position controller17/MATLAB Function ==
  data: u input; y output; t input
function y = fcn(u,t)
%#codegen
if t>u
    y = 1;
else
    y = 0;
end
end

== matlab function first_3phase_multilevel/position controller1/MATLAB Function14 ==
  data: u input; y output; t input
function y = fcn(u,t)
%#codegen
if t>u
    y = 1;
else
    y = 0;
end
end

== matlab function first_3phase_multilevel/position controller17/MATLAB Function3 ==
  data: u input; y output; t input
function y = fcn(u,t)
%#codegen
if t>u
    y = 1;
else
    y = 0;
end
end

== matlab function first_3phase_multilevel/position controller2/MATLAB Function1 ==
  data: u input; y output; t input
function y = fcn(u,t)
%#codegen
if t>u
    y = 1;
else
    y = 0;
end
end

== matlab function first_3phase_multilevel/position controller2/MATLAB Function2 ==
  data: u input; y output; t input
function y = fcn(u,t)
%#codegen
if t>u
    y = 1;
else
    y = 0;
end
end

== matlab function first_3phase_multilevel/position controller1/MATLAB Function15 ==
  data: u input; y output; t input
function y = fcn(u,t)
%#codegen
if t>u
    y = 1;
else
    y = 0;
end
end

== matlab function first_3phase_multilevel/MATLAB Function18 ==
  data: u input; A11 output; time input; B11 output
function [A11,B11] = fcn(u,time)
%#codegen
A11 = u*sin(11*2*pi*50*time);
B11 = u*cos(11*2*pi*50*time);
end

== matlab function first_3phase_multilevel/MATLAB Function19 ==
  data: u input; A5 output; time input; B5 output
function [A5,B5] = fcn(u,time)
%#codegen
A5 = u*sin(5*2*pi*50*time);
B5 = u*cos(5*2*pi*50*time);
end

== matlab function first_3phase_multilevel/MATLAB Function1 ==
  data: u input; A1 output; time input; B1 output
function [A1,B1] = fcn(u,time)
%#codegen
A1 = u*sin(13*2*pi*50*time);
B1 = u*cos(13*2*pi*50*time);
end

== matlab function first_3phase_multilevel/position controller22/MATLAB Function6 ==
  data: u input; y output; t input
function y = fcn(u,t)
%#codegen
if t>u
    y = 1;
else
    y = 0;
end
end

== matlab function first_3phase_multilevel/position controller22/MATLAB Function7 ==
  data: u input; y output; t input; c input
function y = fcn(u,t,c)
%#codegen
if t>u
    y = 1;
else
    y = 0;
end
if c<0.02
    y =0;
end

== matlab function first_3phase_multilevel/MATLAB Function2 ==
  data: u input; A1 output; time input; B1 output
function [A1,B1] = fcn(u,time)
%#codegen
A1 = u*sin(17*2*pi*50*time);
B1 = u*cos(17*2*pi*50*time);
end

== matlab function first_3phase_multilevel/MATLAB Function3 ==
  data: u input; A1 output; time input; B1 output
function [A1,B1] = fcn(u,time)
%#codegen
A1 = u*sin(19*2*pi*50*time);
B1 = u*cos(19*2*pi*50*time);
end

== matlab function first_3phase_multilevel/MATLAB Function10 ==
  data: u input; A1 output; time input; B1 output
function [A1,B1] = fcn(u,time)
%#codegen
A1 = u*sin(19*2*pi*50*time);
B1 = u*cos(19*2*pi*50*time);
end

== matlab function first_3phase_multilevel/position controller3/MATLAB Function15 ==
  data: u input; y output; t input
function y = fcn(u,t)
%#codegen
if t>u
    y = 1;
else
    y = 0;
end
end

== matlab function first_3phase_multilevel/MATLAB Function16 ==
  data: u input; A1 output; time input; B1 output
function [A1,B1] = fcn(u,time)
%#codegen
A1 = u*sin(2*pi*50*time);
B1 = u*cos(2*pi*50*time);
end

== matlab function first_3phase_multilevel/MATLAB Function17 ==
  data: u input; A7 output; time input; B7 output
function [A7,B7] = fcn(u,time)
%#codegen
A7 = u*sin(7*2*pi*50*time);
B7 = u*cos(7*2*pi*50*time);
end

== matlab function first_3phase_multilevel/position controller23/MATLAB Function8 ==
  data: u input; y output; t input
function y = fcn(u,t)
%#codegen
if t>u
    y = 1;
else
    y = 0;
end
end
